simulink model "MPC_Sim"  (R2020a)
settings: Solver=FixedStepAuto  StartTime=0.0  StopTime=100  FixedStep=1e-2  RelTol=1e-3
settings Model: Creator=niran  LastModifiedBy=niran

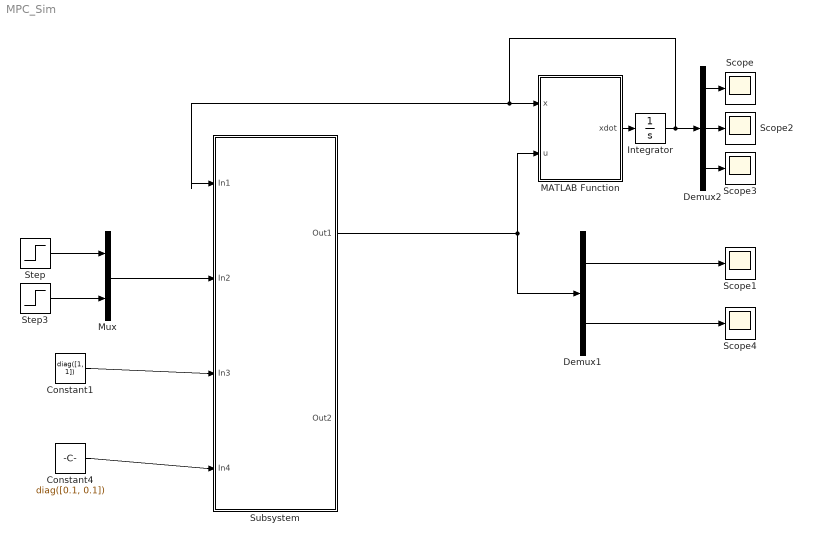
== system MPC_Sim ==
  Constant1 : Constant  Value=diag([1, 1])
  Constant4 : Constant  Value=diag([0.1, 0.1])
  Demux1 : Demux  Outputs=2
  Demux2 : Demux  Outputs=3
  Integrator : Integrator
  MATLAB Function : MATLAB Function  TreatAsAtomicUnit=on
  Mux : Mux  Inputs=2
  Scope{,1..4} (5 alike) : Scope
  Step : Step  Time=50  Before=0.5  SampleTime=0
  Step3 : Step  Time=75  Before=25  After=35  SampleTime=0
  Subsystem : Subsystem  TreatAsAtomicUnit=on  SystemSampleTime=0.1
  wires:
  Demux1/1 -> Scope1/1
  Demux1/2 -> Scope4/1
  MATLAB Function/1(xdot) -> Integrator/1
  Demux2/1 -> Scope/1
  Demux2/2 -> Scope2/1
  Demux2/3 -> Scope3/1
  Step/1 -> Mux/1
  Step3/1 -> Mux/2
  Integrator/1 -> Subsystem/1(In1), MATLAB Function/1(x), Demux2/1
  Subsystem/1(Out1) -> Demux1/1, MATLAB Function/2(u)
  Mux/1 -> Subsystem/2(In2)
  Constant1/1 -> Subsystem/3(In3)
  Constant4/1 -> Subsystem/4(In4)

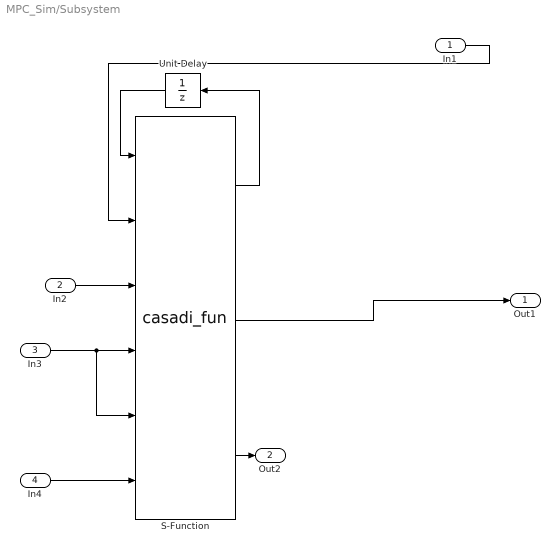
== system MPC_Sim/Subsystem ==
  In1 : Inport
  In2 : Inport  Port=2
  In3 : Inport  Port=3
  In4 : Inport  Port=4
  S-Function : S-Function  FunctionName=casadi_fun  Parameters='MPC_func.casadi', 'MPC_func'  SFunctionDeploymentMode=off  EnableBusSupport=off
  Unit Delay : UnitDelay  SampleTime=-1  HasFrameUpgradeWarning=on
  Out1 : Outport
  Out2 : Outport  Port=2
  wires:
  In3/1 -> S-Function/5, S-Function/4
  In4/1 -> S-Function/6
  Unit Delay/1 -> S-Function/1
  S-Function/3 -> Out2/1
  S-Function/2 -> Out1/1
  S-Function/1 -> Unit Delay/1
  In1/1 -> S-Function/2
  In2/1 -> S-Function/3

== matlab function MPC_Sim/MATLAB Function ==
  data: x input; u input; xdot output
function xdot = fcn(x, u)
    xdot = zeros(3, 1);
    A = [-0.4, 0.1, -2.0;
        0, -0.3, 4.0;
        1.0, 0.0, 0.0];
    B = [1, 1;
        0, 1;
        1, 0];
    
    xdot = A * x + B * u;
end
